simulink model "Mys_P6"  (R2019b)
settings: Solver=VariableStepAuto  StartTime=0.0  StopTime=10  RelTol=1e-3
values from neighbouring files (symbols this model uses):
  b = 0.1    [Tema3_P4.m]    (also in p6_pendulo.m)
  g = 9.8    [p6_pendulo.m]
  I = 0.006    [p6_pendulo.m]
  l = 0.3    [p6_pendulo.m]
  m = 0.2    [p6_pendulo.m]
  M = 0.5    [p6_pendulo.m]
  q = (M+m)*(I+m*l^2)-(m*l)^2    (= 0.0132)    [p6_pendulo.m]
libraries: cstblocks x2, simulink x1
settings Model: Creator=Usuario  LastModifiedBy=Usuario

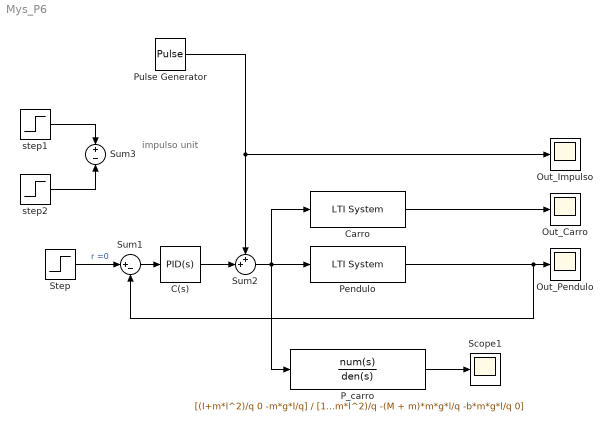
== system Mys_P6 ==
  note: impulso unit
  C(s) : simulink/Continuous/PID Controller  Controller=PID  Form=Parallel  TimeDomain=Continuous-time  SampleTime=-1  IntegratorMethod=Forward Euler  FilterMethod=Forward Euler  ControllerParametersSource=internal  P=100  I=100  D=50  UseFilter=on  N=1000  TunerSelectOption=Transfer Function Based (PID Tuner App)  InitialConditionSource=internal  InitialConditionForIntegrator=0  InitialConditionForFilter=0  DifferentiatorICPrevScaledInput=0  ExternalReset=none  TrackingMode=off  Kt=1  LimitOutput=off  UpperSaturationLimit=inf  LowerSaturationLimit=-inf  LinearizeAsGain=on  AntiWindupMode=none  Kb=1  POutMin=[]  POutMax=[]  IOutMin=[]  IOutMax=[]  DOutMin=[]  DOutMax=[]  NOutMin=[]  NOutMax=[]  SumOutMin=[]  SumOutMax=[]  SaturationOutMin=[]  SaturationOutMax=[]  PParamMin=[]  PParamMax=[]  IParamMin=[]  IParamMax=[]  DParamMin=[]  DParamMax=[]  NParamMin=[]  NParamMax=[]  KbParamMin=[]  KbParamMax=[]  KtParamMin=[]  KtParamMax=[]  KbOutMin=[]  KbOutMax=[]  KtOutMin=[]  KtOutMax=[]  IntegratorOutMin=[]  IntegratorOutMax=[]  FilterOutMin=[]  FilterOutMax=[]  SumI1OutMin=[]  SumI1OutMax=[]  SumI2OutMin=[]  SumI2OutMax=[]  SumI3OutMin=[]  SumI3OutMax=[]  SumI4OutMin=[]  SumI4OutMax=[]  SumDOutMin=[]  SumDOutMax=[]  DifferentiatorOutMin=[]  DifferentiatorOutMax=[]  FilterDiffOutCoefMin=[]  FilterDiffOutCoefMax=[]  ReciprocalOutMin=[]  ReciprocalOutMax=[]  SumDenOutMin=[]  SumDenOutMax=[]  SumNumOutMin=[]  SumNumOutMax=[]  DivideOutMin=[]  DivideOutMax=[]  IntegratorContinuousStateAttributes=''  IntegratorStateMustResolveToSignalObject=off  IntegratorRTWStateStorageClass=Auto  FilterContinuousStateAttributes=''  FilterStateMustResolveToSignalObject=off  FilterRTWStateStorageClass=Auto  ParallelPVariant=InternalParameters  IdealPVariant=Disabled  IVariant=InternalParameters  DVariant=InternalParameters  IntegratorVariant=Continuous  SatVariant=Disabled  AWVariant=Passthrough  PCopyVariant=Disabled  TRVariant=Disabled  FdbkBlocksVariant=Forward  IdealPFdbkVariant=Disabled  SatFdbkVariant=Disabled  DerivativeFilterVariant=ContFilter  NVariant=InternalParameters  NCopyVariant=Disabled  FilterICVariant=InternalICsFilter  IntegratorICVariant=InternalICs  ExternalResetVariant=Disabled  TRSumVariant=Passthrough  SumFdbkVariant=Disabled  SumVariant=Sum_PID
  Carro : cstblocks/LTI System  sys=G2  IC=[]
  Out_Carro : Scope
  Out_Impulso : Scope
  Out_Pendulo : Scope
  P_carro : TransferFcn  Numerator=[(I+m*l^2)/q 0 -m*g*l/q]  Denominator=[1 b*(I + m*l^2)/q -(M + m)*m*g*l/q -b*m*g*l/q 0]
  Pendulo : cstblocks/LTI System  sys=G1  IC=[]
  Pulse Generator : DiscretePulseGenerator  PulseType=Time based  Period=11  PulseWidth=0.1
  Scope1 : Scope
  Step : Step  Time=0  After=0  SampleTime=0
  Sum1 : Sum  Inputs=|+-
  Sum2 : Sum  Inputs=++|
  Sum3 : Sum  Inputs=+|-
  step1 : Step  Time=0  After=1e6  SampleTime=0
  step2 : Step  Time=1/1e6  After=1e6  SampleTime=0
  wires:
  Step/1 -> Sum1/1  "r =0"
  Sum1/1 -> C(s)/1
  C(s)/1 -> Sum2/2
  Sum2/1 -> P_carro/1, Carro/1, Pendulo/1
  Carro/1 -> Out_Carro/1
  Pendulo/1 -> Sum1/2, Out_Pendulo/1
  step1/1 -> Sum3/1
  step2/1 -> Sum3/2
  P_carro/1 -> Scope1/1
  Pulse Generator/1 -> Out_Impulso/1, Sum2/1
